simulink model "Copy_of_sys_PID"  (R2021a)
settings: Solver=FixedStepAuto  StartTime=0.0  StopTime=100  FixedStep=0.02  RelTol=1e-3
undefined symbols (not defined in the file): v, yaw
libraries: simulink x2
(part 2 of 2)

== matlab function Copy_of_sys_PID/Limmitter and Angle//Thrust  ==
  data: F_1 input; F1 output; F_2 input; F2 output; alpha_in_1 input; alpha1 output; alpha_in_2 input; alpha_1_old input; alpha2 output; alpha_flag_out output; alpha_2_old input; F_old_1 input; F_old_2 input; alpha_flag input; sway_flag input; count_sway input; sway_flag output; count_sway output; ref_u_in input; ref_v_in input; turn_above_45_flag input; ref_yaw_old output; turn_above_45_flag_out output; ref_yaw input
function [F1, F2, alpha1, alpha2, alpha_flag_out,sway_flag, count_sway, ref_yaw_old,turn_above_45_flag_out] = fcn(F_1,F_2, alpha_in_1, alpha_in_2, alpha_1_old, alpha_2_old, F_old_1,F_old_2, alpha_flag, sway_flag, count_sway, ref_u_in, ref_v_in, turn_above_45_flag, ref_yaw)
%global alpha_flag

 
    T_max = 1000; % max for trust in both positiv and negativ direction 

  
    %if abs(alpha_in_1) < 7*pi/18 && abs(alpha_in_1) >= 0 
    % sway manuvering (abs(alpha > 70 degrees)) 
    if abs(alpha_in_2) >= 7*pi/18 && abs(alpha_in_2) <= 11*pi/18 || abs(alpha_in_2) <= 25*pi/18 && abs(alpha_in_2) >= 29*pi/18  % manuvering up to 
        
        % limmitter and angle determination
        % angle alpha_2
        % keeps angle between +-180 degrees
        if alpha_in_2 > pi
            alpha_in_2 = alpha_in_2 - 2 * pi;
        elseif alpha_in_2 < -pi
            alpha_in_2 = alpha_in_2 + 2 * pi;
        end       
        % determining the right angle and thrust    
        if alpha_in_2 > pi/2 && alpha_in_2 <= pi% 11*pi/18      %(between 90 and 160 degrees)
            alpha_in_2 = alpha_in_2 - pi;
            F_2 = (-1)*F_2;
        elseif alpha_in_2 < -pi/2 && alpha_in_2 >= -pi% -11*pi/18 %(between -90 and -160 degrees)
            alpha_in_2 = alpha_in_2 + pi;
            F_2 = (-1)*F_2;
        end
        


        % limitter for the thrusters for going sideway
        if abs(F_1) > T_max
            if F_1 < 0
               k_direction = (-1);
            else 
               k_direction = 1;
               
            end
            %F1 = T_max;            
            F1_old = F_1;
            F_1 = T_max*k_direction;
            F_2 = F_1/(F1_old/F_2);   
        %elseif F1 < -T_max
        %    F1 = -T_max;    
        end
        if abs(F_2) > T_max
            if F_2 < 0
               k_direction = (-1);
            else 
               k_direction = 1;
            end
            %F2 = T_max;
            F2_old = F_2;
            F_2 = T_max * k_direction;
            F_1 = F_2/(F2_old/F_1);  
        %elseif F2 < -T_max
        %   F2 = -T_max;    
        end
  
        
        %pod angle limitter (88 degrees)
        if alpha_in_2 >= 22*pi/45 
            alpha_in_2 = 22*pi/45;
        elseif alpha_in_2 <= -22*pi/45 
            alpha_in_2 = -22*pi/45;
        end
        
        % solution for going straight in y direction
%         if alpha_in_1 == 7*pi/18 && alpha_in_2 < 0
%            alpha_in_2 = -alpha_in_2;
%            F_2 = -F_2;
%         end
        
 
        % returning results
        F_1_out = F_1;           
        F_2_out = F_2;
        alpha_out_1 = alpha_in_1;
        alpha_out_2 = alpha_in_2;
        
        
        
        
        
    else % manuuvering alpha less than 70 degrees     
        
        % if F1 is larger than the limit and F2 is positive
        if (F_1 > T_max && abs(F_2) < abs(F_1))
            diff = F_1 - T_max;  

            % if diff is out of range and F_1 > 0
            if ((abs(diff) > T_max)&& ((F_2 > 0) && (((F_2 - diff) > T_max) || (F_2 - diff) < -T_max)) ||  (F_2 < 0) && (((F_2 + diff) > T_max) || (F_2 + diff) < -T_max))             
                F_1_old = F_1;
                F_1 = T_max;
                F_2 = F_1/(F_1_old/F_2);
%                 fprintf("Er HER 1_special")

            elseif (F_2 >= 0)      %F2 is positive
                F_1 = F_1 - diff;
                F_2 = F_2 - diff;
%                 fprintf("Er HER 1_1")
            else                   %F2 is negative
                F_1 = F_1 - diff;
                F_2 = F_2 + diff; 
%                 fprintf("Er HER 1_2")
            end
        end    

        % if F2 is larger than the limit        
        if (F_2 > T_max && abs(F_2) > abs(F_1))          
            diff = F_2 - T_max;  

            % if diff is out of range and F_2 > 0
            if ((abs(diff) > T_max)&& ((F_1 > 0) && (((F_1 - diff) > T_max) || (F_1 - diff) < -T_max)) ||  (F_1 < 0) && (((F_1 + diff) > T_max) || (F_1 + diff) < -T_max))  
                F_2_old = F_2;
                F_2 = T_max;
                F_1 = F_2/(F_2_old/F_1);
%                 fprintf("Er HER 2_special")  

            elseif (F_1 >= 0)      %F1 is positive
                F_1 = F_1 - diff;
                F_2 = F_2 - diff;
%                 fprintf("Er HER 2_1")
            else                   %F1 is negative
                F_1 = F_1 + diff;
                F_2 = F_2 - diff; 
%                 fprintf("Er HER 2_2")
            end
        end

        % if F1 is below the limit
        if (F_1 < -T_max && abs(F_2) < abs(F_1))
            diff = F_1 - (-T_max); 

            % if diff is out of range and F_1 < 0
            if ((abs(diff) > T_max) && ((F_2 > 0) && (((F_2 + diff) > T_max) || (F_2 + diff) < -T_max)) ||  (F_2 < 0) && (((F_2 - diff) > T_max) || (F_2 - diff) < -T_max))  
                F_1_old = F_1;
                F_1 = -T_max;
                F_2 = F_1/(F_1_old/F_2);
%                 fprintf("Er HER 3_special")

            elseif (F_2 >= 0)      %F2 is positive
                F_1 = F_1 - diff;
                F_2 = F_2 + diff;
%                 fprintf("Er HER 3_1")
            else                   %F2 is negattive
                F_1 = F_1 - diff;
                F_2 = F_2 - diff;
%                 fprintf("Er HER 3_2")
            end
        end

        % if F2 is below the limit
        if (F_2 < -T_max && abs(F_2) > abs(F_1))
            diff = F_2 - (-T_max);

            % if diff is out of range and F_2 < 0
            if ((abs(diff) > T_max) && ((F_1 > 0) && (((F_1 - diff) > T_max) || (F_1 - diff) < -T_max)) ||  (F_1 < 0) && (((F_1 + diff) > T_max) || (F_2 + diff) < -T_max))  
                F_2_old = F_2;
                F_2 = -T_max;
                F_1 = F_2/(F_2_old/F_1);
%                 fprintf("Er HER 4_special")

            elseif (F_1 >= 0)     %F1 is positive
                F_1 = F_1 + diff;
                F_2 = F_2 - diff;
%                 fprintf("Er HER 4_1")
            else                  %F1 is negative
                F_1 = F_1 - diff;
                F_2 = F_2 - diff;    
%                 fprintf("Er HER 4_2")
            end
        end



        % angle alfa 
        % between +-180 degrees
        if alpha_in_1 > pi 
            alpha_in_1 = alpha_in_1 - 2 * pi;
        elseif alpha_in_1 < -pi 
            alpha_in_1 = alpha_in_1 + 2 * pi;
        end      
%         fprintf("alpha = ")
%         disp(alpha_in_1)
%         fprintf("F1 = ")
%         disp(F_1)
        % determining the right angle and thrust    
        if alpha_in_1 > pi/2       %(above 90 degrees)
            alpha_out = alpha_in_1 - pi;
            F_1_out = (-1)*F_1;
            F_2_out = (-1)*F_2;
%             fprintf("1-------- alpha>pi/2 ---------")
        elseif alpha_in_1 < -pi/2  %(below -90 degrees)
            alpha_out = alpha_in_1 + pi;
            F_1_out = (-1)*F_1;
            F_2_out = (-1)*F_2;
%             %fprintf("2-------- alpha<pi/2 ---------")
            
%         if alpha_in_1 > pi/2
%             alpha_out = alpha_in_1 - (2*pi);
%             F_1_out = (-1)*F_1;
%             F_2_out = (-1)*F_2;
% 
%         elseif alpha_in_1 < -pi/2
%             alpha_out = alpha_in_1 + 180;
%             F_1_out = (-1)*F_1;
%             F_2_out = (-1)*F_2;

        else 
            alpha_out = alpha_in_1;
            F_1_out = F_1;
            F_2_out = F_2;
        end
       
        alpha_out_1 = alpha_out;
        alpha_out_2 = alpha_out_1;
     
    end
    
    
 
    disp("ALpha muligløsnng:")  
    disp(alpha_out_1)
    disp(alpha_out_2)
    
    
    
    %|| (abs(u_con_sig)<abs(v_con_sig) && ref_v_in == 0)
    
    
    
    % stops, turns and keep motor values    
    if ( (((alpha_out_2 > 0 && alpha_2_old < 0) || (alpha_out_2 < 0 && alpha_2_old > 0)) && abs(alpha_out_2 - alpha_2_old )> 7*pi/18 ) ||  (alpha_flag == 1)  || (sway_flag == 1) ) % Forces to 0 and turneing the pods (larger X Degrees)
        %(acos(complex(abs(ref_u_in)/abs(ref_v_in))) < 5*pi/12) ||
        %(atan((abs(ref_u_in)/abs(ref_v_in))) > 5*pi/12)  ||
        disp("####################### stop motor #####################")
    %if abs(alpha_out_2 - alpha_2_old )> 7*pi/18 || (alpha_out_2 > 0 && alpha_2_old < 0) || (alpha_out_2 < 0 && alpha_2_old > 0) ||  alpha_flag == 1 % Forces to 0 and turneing the pods (larger X Degrees)
        %alpha_flag = 1;
        %turn_yes = 0;
        %if abs(alpha_out_2 - alpha_2_old) > pi/4 || (alpha_out_2 > 0 && alpha_2_old < 0) || (alpha_out_2 < 0 && alpha_2_old > 0)
 
        if ((sway_flag == 0) && alpha_flag ==1 )
            disp("Venter på podvinkel");
%             disp(alpha_2_old)
%             disp(alpha_out_2)
%             disp(alpha_out_2-alpha_2_old)
%             disp("-------slukket::::::::::---------_________::::::::::::::")
            F_1_out = 0;
            F_2_out = 0;
            F_old_1 = F_1;
            F_old_2 = F_2;
         else
            F_1_out = F_1;
            F_2_out = F_2; 
            
         end
         turn_yes = 0;
         alpha_flag = 1;
%             alpha_1 = alpha_1;
%             alpha_2 = alpha_2;
        %else
            %alpha_flag=0;
%          end
%          if abs(abs(alpha_out_2) - abs(alpha_2_old)) < 0.2 %pi/18 
%             F1 = F1;
%             F2 = F2;
%             alpha_1 = alpha_1;
%             alpha_2 = alpha_2;
            

         if ((abs(alpha_out_2 - alpha_2_old) < 0.01) && sway_flag == 0)
               %pi/18
               alpha_flag = 0;
               turn_yes = 1;
               fprintf("indenfor x grader");
%                disp(alpha_2_old)
%                disp(alpha_out_2)
%          else
%              disp("Venter på podvinkel");
%              disp(alpha_2_old)
%              disp(alpha_out_2)
%              disp(alpha_out_2-alpha_2_old)
% %            F_1_out = 0;
% %            F_2_out = 0;


          end
            
           
          %|| (ref_v_in == 0 && abs(v_con_sig) > abs(u_con_sig))  
          if (((turn_yes == 1) || (sway_flag == 1)) &&  (abs(atan(((ref_v_in)/(ref_u_in)))) > 5*pi/12) )% keeps the velocity/thrust 5*pi/12
               
               disp("###### Holde værdi#####")
               sway_flag = 1;
               count_sway = count_sway + 1;
               disp("_-_-_-_-_- counter =")
               disp(count_sway)
               
           
                   
%                F_1_out = F_1; % returning F_1
%                F_2_out = F_2; % returning F_1
%                alpha_out_1 = alpha_in_1; % returning input from when the flag was set
%                alpha_out_2 = alpha_in_2; % returning input from when the flag was set
                
               F_1_out = F_old_1; % returning F_1
               F_2_out = F_old_2; % returning F_1
%                disp("akpha førrrrr =")
%                disp(alpha_out_1)
               alpha_out_1 = alpha_1_old; % returning input from when the flag was set
               alpha_out_2 = alpha_2_old; % returning input from when the flag was set
               disp("alpha holde konstant")
               disp(alpha_out_1)
               disp(alpha_out_2)
               
%                disp("-------turn_Sway_flag::::::::::---------_________::::::::::::::")
                
               if count_sway >= 6/0.02 %(2sec 50Hz 5 sec 10Hz) %stops counter and goes on
                   sway_flag = 0;
                   
                   count_sway = 0;

                   turn_yes = 0;
                   alpha_flag =0;
                  
               
               
                   disp("_________________% SEK overstået_____________-------------------_________::::::::::::::::")

               end
                  
        
       
            
          end
             
            
            
        %end
%         disp("ALPHA_FLAG =");
%         disp(alpha_flag)
    end
%         disp("ALPHA_FLAG =");
%         disp(alpha_flag)    


disp("alpha_out end")
disp(alpha_out_1)
disp(alpha_out_2)

% disp('LIMITER F1 -_-----------------------------------');
% disp(F_1_out);
        
        
turn_above_45_flag_out = turn_above_45_flag;     
ref_yaw_old = ref_yaw;            
F1 = F_1_out;
F2 = F_2_out;
alpha1 = alpha_out_1;
alpha2 = alpha_out_2;
alpha_flag_out = alpha_flag;

== matlab function Copy_of_sys_PID/Turn overwrite (orientation) ==
  data: ref_u input; ref_u_out output; ref_v input; ref_yaw input; yaw_USV input; ref_v_out output; ref_yaw_out output; turn_above_45_flag input; turn_above_45_flag_out output; rot_thrust input; rot_thrust_out output; count_cnt input; count_cnt_o output
function [ref_u_out,ref_v_out, ref_yaw_out, turn_above_45_flag_out, rot_thrust_out,count_cnt_o] = fcn(ref_u,ref_v, ref_yaw, yaw_USV, turn_above_45_flag, rot_thrust,count_cnt)

        if (ref_yaw < yaw_USV)
            direction = -1;
        elseif(ref_yaw > yaw_USV)
            direction = 1;
        else
            direction = 0;
        end
        
        
      
    if ((abs(ref_yaw - yaw_USV) > 0.2) && (abs(ref_v)>=abs(ref_u)) || turn_above_45_flag == 1)
        turn_above_45_flag_out = 1;
%         if(abs(ref_yaw) < 0.01)
%             ref_u_out = ref_u;  
%             ref_v_out = ref_v;
%             ref_yaw_out =  0;
%             
%         else
            
            ref_u_out = 0;  
            ref_v_out = 0;
            %ref_yaw_out = ref_yaw; % Yaw_USV

            ref_yaw_out =  (yaw_USV + 0.2*direction)
        %disp("FFFFFFFFFFFFFFFFFFFFFFFFFFFFFFFFFFFFFFFFFFF")
        
%         count_cnt = count_cnt+1;
%         if count_cnt >= 0/0.02 %(2sec 50Hz 5 sec 10Hz) %stops counter and goes on                  
%             ref_yaw_out =  (yaw_USV + 0.05*direction); %ref_yaw; 
         %end
        
        
        
        if (abs(ref_yaw - yaw_USV) < 0.01)
             turn_above_45_flag_out = 0;
             count_cnt = 0;
        end
        
    else 
        ref_u_out = ref_u;  
        ref_v_out = ref_v;
        ref_yaw_out = ref_yaw;
        %disp("KKKKKKKKKKKKKKKKKKKKKKKKKKKKKKKKKKKKKKKKK")
        turn_above_45_flag_out = 0;
        count_cnt = 0;
    end
   
    rot_thrust_out = rot_thrust;
    count_cnt_o = count_cnt;

== matlab function Copy_of_sys_PID/PID Controllers/PIDs/MATLAB Function2 ==
  data: ref_u input; y output; ref_v input
function y = fcn(ref_u,ref_v)

%     if (ref_v == 0)
%         ref_v = 0.00001;
%     end
%     if (ref_u == 0)
%         ref_u = 0.00001;
%     end
%     
    

%     if(abs(ref_u)<0.1)
%         y = 1;
%         
    %if(abs(atan(complex(abs(ref_u)/abs(ref_v)))) < pi/4)
    if(abs(atan(((ref_v)/(ref_u)))) > pi/4)
        y = 1;
    else
        y = 0;
    end
    
disp("___________yyyy________________")
disp(y)
disp(abs(atan(complex(ref_u/ref_v))))

== matlab function Copy_of_sys_PID/MATLAB Function ==
  data: u input; y output
function y = fcn(u)
   if(u == 0.0)
        out = 0.00000000000000000001;
    else
        out = u;
    
    end
    
    
  

y = out;
